simulink model "rotor_sim"  (Simulink 7.7)
settings: Solver=ode4  StartTime=0.0  StopTime=3  FixedStep=1/25  RelTol=1e-3
PostLoadFcn:
  | bus_RotorParameters;
  | bus_FuselageParameters;
  | bus_FinParameters;
  | bus_GeometryParameters;
  | bus_Environment;
libraries: simulink x4, UAVdesign_net x1
settings Model: Creator=Emanuel  LastModifiedBy=Emanuel
settings DebuggingCC: StrictBusMsg=Warning
settings SFSimCC: SimParseCustomCode=off

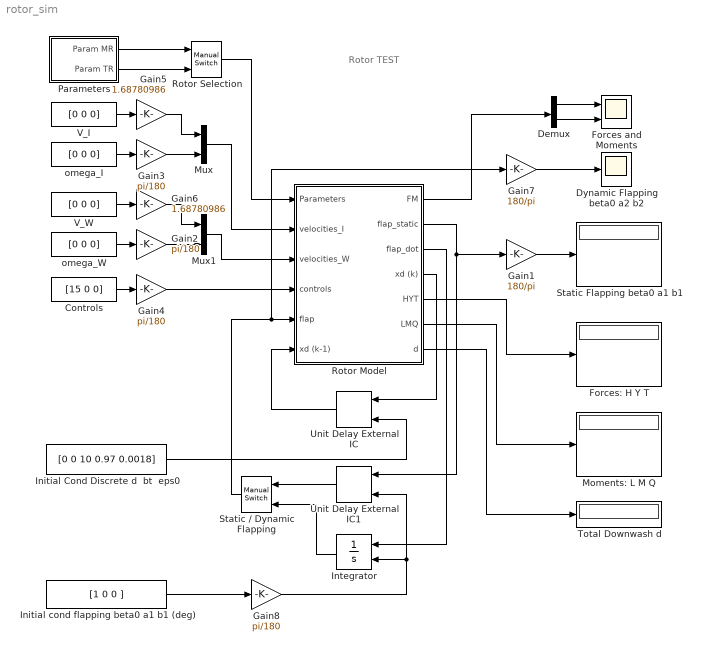
== system rotor_sim ==
  note: Rotor TEST
  Controls : Constant  Value=[15 0 0]
  Demux : Demux  Outputs=[3 3]
  Dynamic Flapping beta0 a2 b2 : Scope
      settings: YMin=-10  YMax=10
  Forces and Moments : Scope  NumInputPorts=2
      settings: YMin=-6000~-10000  YMax=2000~10000
  Forces: H Y T : Display
  Gain1 : Gain  Gain=180/pi
  Gain{2..4,8} (4 alike) : Gain  Gain=pi/180
  Gain5 : Gain  Gain=1.68780986
  Gain6 : Gain  Gain=1.68780986
  Gain7 : Gain  Gain=180/pi
  Initial Cond Discrete d  bt  eps0 : Constant  Value=[0 0 10 0.97 0.0018]
  Initial cond flapping beta0 a1 b1 (deg) : Constant  Value=[1 0 0 ]
  Integrator : Integrator  InitialConditionSource=external
  Moments: L M Q : Display
  Mux : Mux  Inputs=2
  Mux1 : Mux  Inputs=2
  Parameters : Subsystem
      settings: OpenFcn=gui_HelicopterParameters( 'Block', [get_param(gcb, 'Parent') '/' get_param(gcb, 'Name')]);
  Rotor Model : Subsystem
  Rotor Selection : simulink/Signal Routing/Manual Switch  SystemSampleTime=-1  sw=1  action=0  varsize=off
  Static / Dynamic Flapping : simulink/Signal Routing/Manual Switch  SystemSampleTime=-1  sw=1  action=0  varsize=off
  Static Flapping beta0 a1 b1 : Display
  Total Downwash d : Display
  Unit Delay External IC : simulink/Additional Math & Discrete/Additional Discrete/Unit Delay External IC  SystemSampleTime=-1  tsamp=1/25
  Unit Delay External IC1 : simulink/Additional Math & Discrete/Additional Discrete/Unit Delay External IC  SystemSampleTime=-1  tsamp=1/25
  V_I : Constant  Value=[0 0 0]
  V_W : Constant  Value=[0 0 0]
  omega_I : Constant  Value=[0 0 0]
  omega_W : Constant  Value=[0 0 0]
  wires:
  Unit Delay External IC/1 -> Rotor Model/6(xd (k-1))
  Rotor Model/4(xd (k)) -> Unit Delay External IC/1
  Initial Cond Discrete d  bt  eps0/1 -> Unit Delay External IC/2
  Rotor Model/3(flap_dot) -> Integrator/1
  Initial cond flapping beta0 a1 b1 (deg)/1 -> Gain8/1
  Controls/1 -> Gain4/1
  V_I/1 -> Gain5/1
  omega_I/1 -> Gain3/1
  Mux/1 -> Rotor Model/2(velocities_I)
  Rotor Model/1(FM) -> Demux/1
  Gain1/1 -> Static Flapping beta0 a1 b1/1
  Rotor Model/2(flap_static) -> Gain1/1, Unit Delay External IC1/1
  V_W/1 -> Gain6/1
  omega_W/1 -> Gain2/1
  Mux1/1 -> Rotor Model/3(velocities_W)
  Gain2/1 -> Mux1/2
  Gain3/1 -> Mux/2
  Gain4/1 -> Rotor Model/4(controls)
  Rotor Model/5(HYT) -> Forces: H Y T/1
  Rotor Model/6(LMQ) -> Moments: L M Q/1
  Rotor Model/7(d) -> Total Downwash d/1
  Gain6/1 -> Mux1/1
  Gain5/1 -> Mux/1
  Integrator/1 -> Static / Dynamic Flapping/2
  Static / Dynamic Flapping/1 -> Rotor Model/5(flap), Gain7/1
  Unit Delay External IC1/1 -> Static / Dynamic Flapping/1
  Demux/1 -> Forces and Moments/1
  Demux/2 -> Forces and Moments/2
  Gain7/1 -> Dynamic Flapping beta0 a2 b2/1
  Gain8/1 -> Integrator/2, Unit Delay External IC1/2
  Parameters/1(Param MR) -> Rotor Selection/1
  Parameters/2(Param TR) -> Rotor Selection/2
  Rotor Selection/1 -> Rotor Model/1(Parameters)

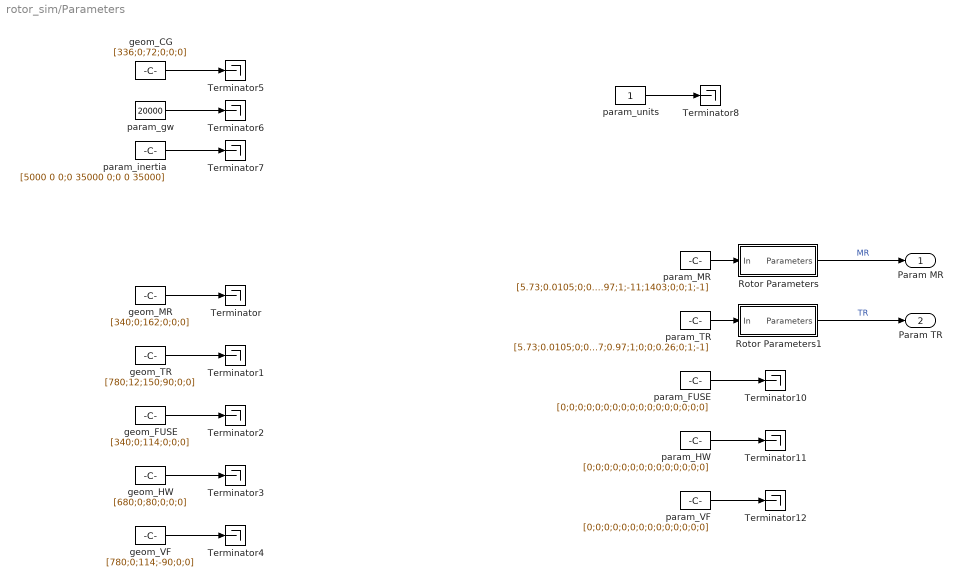
== system rotor_sim/Parameters ==
  Rotor Parameters : Subsystem
  Rotor Parameters1 : Subsystem
  Terminator{,1..8,10..12} (12 alike) : Terminator
  geom_CG : Constant  Value=[336;0;72;0;0;0]
  geom_FUSE : Constant  Value=[340;0;114;0;0;0]
  geom_HW : Constant  Value=[680;0;80;0;0;0]
  geom_MR : Constant  Value=[340;0;162;0;0;0]
  geom_TR : Constant  Value=[780;12;150;90;0;0]
  geom_VF : Constant  Value=[780;0;114;-90;0;0]
  param_FUSE : Constant  Value=[0;0;0;0;0;0;0;0;0;0;0;0;0;0;0;0;0]
  param_HW : Constant  Value=[0;0;0;0;0;0;0;0;0;0;0;0;0;0]
  param_MR : Constant  Value=[5.73;0.0105;0;0.01325;0;0;0;0;2;22;2;0.97;0.97;1;-11;1403;0;0;1;-1]
  param_TR : Constant  Value=[5.73;0.0105;0;0.01325;0;-45;0;0;4;6.5;1.25;0.97;0.97;1;0;0;0.26;0;1;-1]
  param_VF : Constant  Value=[0;0;0;0;0;0;0;0;0;0;0;0;0;0]
  param_gw : Constant  Value=20000
  param_inertia : Constant  Value=[5000 0 0;0 35000 0;0 0 35000]
  param_units : Constant
  Param MR : Outport
  Param TR : Outport  Port=2
  wires:
  geom_MR/1 -> Terminator/1
  geom_TR/1 -> Terminator1/1
  geom_FUSE/1 -> Terminator2/1
  geom_HW/1 -> Terminator3/1
  geom_VF/1 -> Terminator4/1
  param_MR/1 -> Rotor Parameters/1(In)
  param_TR/1 -> Rotor Parameters1/1(In)
  param_FUSE/1 -> Terminator10/1
  param_VF/1 -> Terminator12/1
  param_HW/1 -> Terminator11/1
  geom_CG/1 -> Terminator5/1
  param_gw/1 -> Terminator6/1
  param_inertia/1 -> Terminator7/1
  param_units/1 -> Terminator8/1
  Rotor Parameters1/1(Parameters) -> Param TR/1  "TR"
  Rotor Parameters/1(Parameters) -> Param MR/1  "MR"

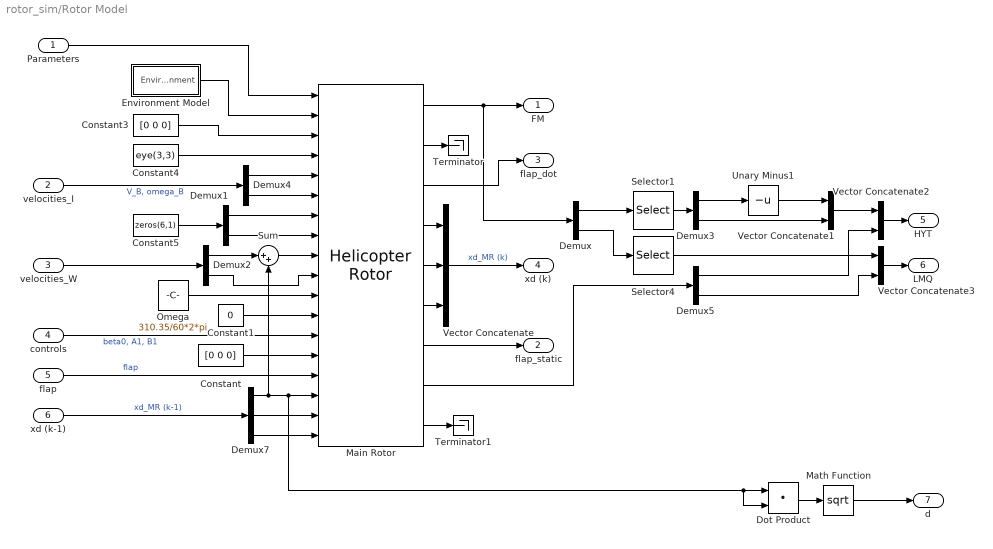
== system rotor_sim/Rotor Model ==
  Parameters : Inport  OutDataTypeStr=Bus: RotorParameters
  velocities_I : Inport  Port=2
  velocities_W : Inport  Port=3
  controls : Inport  Port=4
  flap : Inport  Port=5
  xd (k-1) : Inport  Port=6
  Constant : Constant  Value=[0 0 0]
  Constant1 : Constant  Value=0
  Constant3 : Constant  Value=[0 0 0]
  Constant4 : Constant  Value=eye(3,3)
  Constant5 : Constant  Value=zeros(6,1)
  Demux{,1..5} (6 alike) : Demux  Outputs=2
  Demux7 : Demux  Outputs=[3 1 1]
  Dot Product : DotProduct  InputSameDT=on  OutDataTypeStr=Inherit: Inherit via internal rule
  Environment Model : Subsystem
  Main Rotor : UAVdesign_net/Subsystem Models/Helicopter Rotor  SystemSampleTime=-1
  Math Function : Math  Operator=sqrt  SaturateOnIntegerOverflow=on
  Omega : Constant  Value=310.35/60*2*pi
  Selector1 : Selector  InputPortWidth=3  IndexOptions=Index vector (dialog)  Indices=[1 2]  OutputSizes=1
  Selector4 : Selector  InputPortWidth=3  IndexOptions=Index vector (dialog)  Indices=[1 2]  OutputSizes=1
  Sum : Sum  Inputs=|++
  Terminator : Terminator
  Terminator1 : Terminator
  Unary Minus1 : UnaryMinus
  Vector Concatenate : Concatenate  NumInputs=3  Mode=Vector
  Vector Concatenate1 : Concatenate  Mode=Vector
  Vector Concatenate2 : Concatenate  Mode=Vector
  Vector Concatenate3 : Concatenate  Mode=Vector
  FM : Outport
  flap_static : Outport  Port=2
  flap_dot : Outport  Port=3
  xd (k) : Outport  Port=4
  HYT : Outport  Port=5
  LMQ : Outport  Port=6
  d : Outport  Port=7
  wires:
  Main Rotor/1 -> FM/1, Demux/1
  Demux4/1 -> Main Rotor/5
  Demux4/2 -> Main Rotor/6
  Demux1/1 -> Main Rotor/7
  Demux1/2 -> Main Rotor/8
  Constant/1 -> Main Rotor/14
  Constant1/1 -> Main Rotor/12
  Omega/1 -> Main Rotor/11
  controls/1 -> Main Rotor/13  "beta0, A1, B1"
  Parameters/1 -> Main Rotor/1
  velocities_I/1 -> Demux4/1  "V_B, omega_B"
  flap/1 -> Main Rotor/15  "flap"
  Demux7/2 -> Main Rotor/17
  Demux7/3 -> Main Rotor/18
  xd (k-1)/1 -> Demux7/1  "xd_MR (k-1)"
  Vector Concatenate/1 -> xd (k)/1  "xd_MR (k)"
  Constant3/1 -> Main Rotor/3
  Constant4/1 -> Main Rotor/4
  Environment Model/1(Environment) -> Main Rotor/2
  Constant5/1 -> Demux1/1
  Demux7/1 -> Sum/2, Main Rotor/16, Dot Product/1, Dot Product/2
  Sum/1 -> Main Rotor/9
  Demux2/1 -> Sum/1
  Demux2/2 -> Main Rotor/10
  velocities_W/1 -> Demux2/1
  Demux/1 -> Selector1/1
  Demux/2 -> Selector4/1
  Dot Product/1 -> Math Function/1
  Math Function/1 -> d/1
  Selector1/1 -> Demux3/1
  Vector Concatenate2/1 -> HYT/1
  Vector Concatenate3/1 -> LMQ/1
  Selector4/1 -> Vector Concatenate3/1
  Demux5/1 -> Vector Concatenate2/2
  Vector Concatenate1/1 -> Vector Concatenate2/1
  Unary Minus1/1 -> Vector Concatenate1/1
  Demux3/1 -> Unary Minus1/1
  Demux3/2 -> Vector Concatenate1/2
  Main Rotor/7 -> flap_static/1
  Main Rotor/4 -> Vector Concatenate/1
  Main Rotor/5 -> Vector Concatenate/2
  Main Rotor/6 -> Vector Concatenate/3
  Main Rotor/3 -> flap_dot/1
  Main Rotor/8 -> Demux5/1
  Demux5/2 -> Vector Concatenate3/2
  Main Rotor/2 -> Terminator/1
  Main Rotor/9 -> Terminator1/1

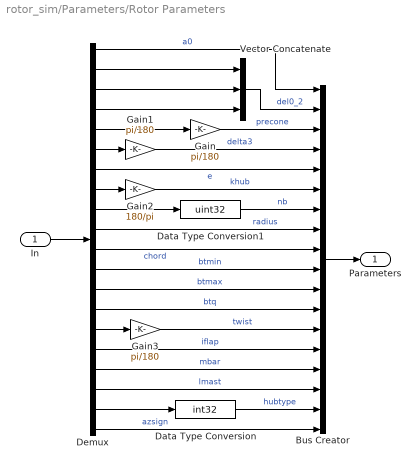
== system rotor_sim/Parameters/Rotor Parameters ==
  In : Inport
  Bus Creator : BusCreator  Inputs=18  OutDataTypeStr=Bus: RotorParameters  NonVirtualBus=on
  Data Type Conversion : DataTypeConversion  OutDataTypeStr=int32  RndMeth=Nearest
  Data Type Conversion1 : DataTypeConversion  OutDataTypeStr=uint32  RndMeth=Nearest
  Demux : Demux  Outputs=20
  Gain : Gain  Gain=pi/180
  Gain1 : Gain  Gain=pi/180
  Gain2 : Gain  Gain=180/pi
  Gain3 : Gain  Gain=pi/180
  Vector Concatenate : Concatenate  NumInputs=3  Mode=Vector
  Parameters : Outport  OutDataTypeStr=Bus: RotorParameters
  wires:
  Demux/14 -> Bus Creator/12  "btq"
  Demux/15 -> Gain3/1
  Demux/12 -> Bus Creator/10  "btmin"
  Demux/11 -> Bus Creator/9  "chord"
  Demux/10 -> Bus Creator/8  "radius"
  Demux/9 -> Data Type Conversion1/1
  Data Type Conversion1/1 -> Bus Creator/7  "nb"
  Demux/8 -> Gain2/1
  Demux/7 -> Bus Creator/5  "e"
  Demux/6 -> Gain1/1
  Demux/5 -> Gain/1
  Gain3/1 -> Bus Creator/13  "twist"
  Gain2/1 -> Bus Creator/6  "khub"
  Gain1/1 -> Bus Creator/4  "delta3"
  Gain/1 -> Bus Creator/3  "precone"
  Demux/19 -> Data Type Conversion/1
  Data Type Conversion/1 -> Bus Creator/17  "hubtype"
  In/1 -> Demux/1
  Vector Concatenate/1 -> Bus Creator/2  "del0_2"
  Demux/2 -> Vector Concatenate/1
  Demux/3 -> Vector Concatenate/2
  Demux/4 -> Vector Concatenate/3
  Bus Creator/1 -> Parameters/1
  Demux/1 -> Bus Creator/1  "a0"
  Demux/13 -> Bus Creator/11  "btmax"
  Demux/16 -> Bus Creator/14  "iflap"
  Demux/17 -> Bus Creator/15  "mbar"
  Demux/18 -> Bus Creator/16  "lmast"
  Demux/20 -> Bus Creator/18  "azsign"

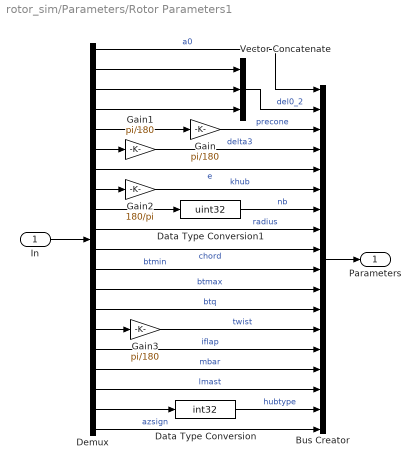
== system rotor_sim/Parameters/Rotor Parameters1 ==
  In : Inport
  Bus Creator : BusCreator  Inputs=18  OutDataTypeStr=Bus: RotorParameters  NonVirtualBus=on
  Data Type Conversion : DataTypeConversion  OutDataTypeStr=int32  RndMeth=Nearest
  Data Type Conversion1 : DataTypeConversion  OutDataTypeStr=uint32  RndMeth=Nearest
  Demux : Demux  Outputs=20
  Gain : Gain  Gain=pi/180
  Gain1 : Gain  Gain=pi/180
  Gain2 : Gain  Gain=180/pi
  Gain3 : Gain  Gain=pi/180
  Vector Concatenate : Concatenate  NumInputs=3  Mode=Vector
  Parameters : Outport  OutDataTypeStr=Bus: RotorParameters
  wires:
  Demux/20 -> Bus Creator/18  "azsign"
  Demux/18 -> Bus Creator/16  "lmast"
  Demux/17 -> Bus Creator/15  "mbar"
  Demux/16 -> Bus Creator/14  "iflap"
  Demux/13 -> Bus Creator/11  "btmax"
  Demux/1 -> Bus Creator/1  "a0"
  Bus Creator/1 -> Parameters/1
  Demux/4 -> Vector Concatenate/3
  Demux/3 -> Vector Concatenate/2
  Demux/2 -> Vector Concatenate/1
  Vector Concatenate/1 -> Bus Creator/2  "del0_2"
  In/1 -> Demux/1
  Data Type Conversion/1 -> Bus Creator/17  "hubtype"
  Demux/19 -> Data Type Conversion/1
  Gain/1 -> Bus Creator/3  "precone"
  Gain1/1 -> Bus Creator/4  "delta3"
  Gain2/1 -> Bus Creator/6  "khub"
  Gain3/1 -> Bus Creator/13  "twist"
  Demux/5 -> Gain/1
  Demux/6 -> Gain1/1
  Demux/7 -> Bus Creator/5  "e"
  Demux/8 -> Gain2/1
  Data Type Conversion1/1 -> Bus Creator/7  "nb"
  Demux/9 -> Data Type Conversion1/1
  Demux/10 -> Bus Creator/8  "radius"
  Demux/11 -> Bus Creator/9  "chord"
  Demux/12 -> Bus Creator/10  "btmin"
  Demux/15 -> Gain3/1
  Demux/14 -> Bus Creator/12  "btq"

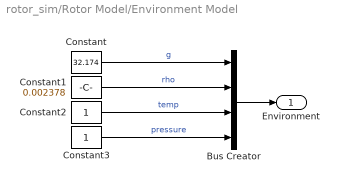
== system rotor_sim/Rotor Model/Environment Model ==
  Bus Creator : BusCreator  OutDataTypeStr=Bus: Environment  NonVirtualBus=on
  Constant : Constant  Value=32.174
  Constant1 : Constant  Value=0.002378
  Constant2 : Constant
  Constant3 : Constant
  Environment : Outport  OutDataTypeStr=Bus: Environment
  wires:
  Bus Creator/1 -> Environment/1
  Constant/1 -> Bus Creator/1  "g"
  Constant1/1 -> Bus Creator/2  "rho"
  Constant2/1 -> Bus Creator/3  "temp"
  Constant3/1 -> Bus Creator/4  "pressure"
